simulink model "dspddc"  (Simulink 8.3)
settings: Solver=FixedStepDiscrete  SolverMode=SingleTasking  StartTime=0.0  StopTime=20500/69.333e6  RelTol=1e-3
model workspace (MATLAB code in the model file):
  | gsmcoeffs
libraries: dspmlti4 x4, simulink x2, dspsigops x2, dspsrcs4 x1, dspmisc x1
settings Model: MinMaxOverflowLogging=OverflowOnly  Creator=The MathWorks Inc.  ExtModeAutoUpdateStatusClock=off
settings DataIOCC: LimitDataPoints=off  SaveOutput=off  SaveTime=off  SignalLoggingName=sigsOut
settings OptimizationCC: InlineParams=on  InlineInvariantSignals=on  ExpressionDepthLimit=2147483647  InitFltsAndDblsToZero=on  EfficientMapNaN2IntZero=off
settings DebuggingCC: SaveWithParameterizedLinksMsg=none  CheckExecutionContextPreStartOutputMsg=on  CheckExecutionContextRuntimeOutputMsg=on  SignalResolutionControl=TryResolveAllWithWarning  SolverPrmCheckMsg=none  InheritedTsInSrcMsg=none  MultiTaskDSMMsg=warning  MultiTaskCondExecSysMsg=none  IntegerOverflowMsg=none  ParameterPrecisionLossMsg=none  FcnCallInpInsideContextMsg=UseLocalSettings  StrictBusMsg=None
settings HardwareCC: ProdHWDeviceType=ASIC/FPGA  ProdEqTarget=off
settings RTWCC: IncludeERTFirstTime=on
settings GRTTargetCC: TargetFcnLib=ansi_tfl_tmw.mat

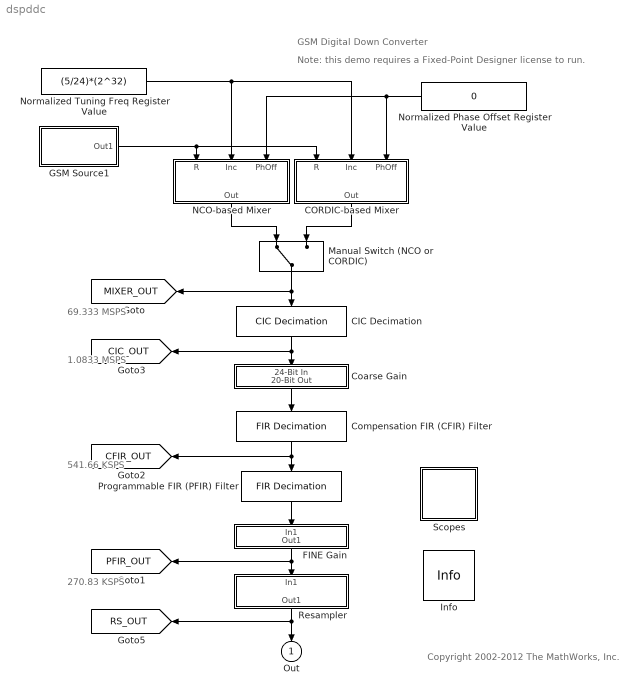
== system dspddc ==
  note: 1.0833
      | MSPS
  note: 541.66
      | KSPS
  note: 270.83
      | KSPS
  note: 69.333
      | MSPS
  note: GSM Digital Down Converter
  note: Note: this demo requires a Fixed-Point Designer license to run.
  note: Copyright 2002-2012 The MathWorks, Inc.
  CIC Decimation : dspmlti4/CIC Decimation  filtFrom=Dialog  filtobj=Hm_decim  ftype=Decimator  R=64  M=1  N=5  filterInternals=Minimum section word lengths  BPS=[50 29 24 24 24 24 24 24 24 24]  FLPS=0  outputWordLength=24  outputFracLength=0  launchFVT=off  framing=Maintain input frame rate  RateOptions=Allow multirate processing
  CORDIC-based Mixer : Subsystem
  Coarse Gain : Subsystem  mask(Coarse Gain){coarse_gain=0}
      mask prompts: coarse_gain "COARSE gain (0-7):"
      mask Help: web(dspdhelp, '-helpbrowser');
      mask Display: disp('Coarse Gain')
  Compensation FIR (CFIR) Filter : dspmlti4/FIR Decimation  h=cfir  D=2  filtStruct=Direct form  framing=Maintain input frame size  inputOffset=0  outputBufInitCond=0  firstCoeffMode=Specify word length  firstCoeffWordLength=16  firstCoeffFracLength=0  firstCoeffDataTypeStr=fixdt(1,16)  firstCoeffLastDataTypeStr=fixdt(1,16)  firstCoeffMin=[]  firstCoeffMax=[]  outputMode=Binary point scaling  outputWordLength=20  outputFracLength=-12  outputDataTypeStr=fixdt(1,20,-12)  outputLastDataTypeStr=fixdt(1,20,-12)  outputMin=[]  outputMax=[]  roundingMode=Floor  overflowMode=off  FilterSource=Specify via dialog  FilterObject=Hm_firdecim
  FINE Gain : Subsystem  mask(Fine Gain){g=1024}
      mask prompts: g "FINE gain (1-16383):"
      mask help: Valid FINE (gain parameter) inputs are positive integers less than 16383. The FINE_GAIN is calculated as FINE/1024.
      mask Help: web(dspdhelp, '-helpbrowser');
      mask Display: disp('Fine Gain')
  GSM Source1 : Subsystem  mask(GSM Source){source_type=Chirp}
      mask prompts: source_type "Source type:"
      mask init:
      | pure_tune_input = (source_type - 1);
      mask Help: web(dspdhelp, '-helpbrowser');
      mask TypeOptions source_type: Chirp | Sinusoid
      mask Display:
      | disp(['GSM' 10 'Source']);
      | 
      | 
      | 
      | 
      | 
      | 
      | port_label('output', 1, 'A/D');
  Info : dspmisc/Info  SystemSampleTime=-1
  Manual Switch (NCO or CORDIC) : ManualSwitch
  NCO-based Mixer : Subsystem
  Normalized Phase Offset Register Value : Constant  Value=0  OutDataTypeStr=int16  SampleTime=-1
  Normalized Tuning Freq Register Value : Constant  Value=(5/24)*(2^32)  OutDataTypeStr=int32
  Programmable FIR (PFIR) Filter : dspmlti4/FIR Decimation  h=pfir  D=2  filtStruct=Direct form  framing=Maintain input frame size  inputOffset=0  outputBufInitCond=0  firstCoeffMode=Specify word length  firstCoeffWordLength=16  firstCoeffFracLength=0  firstCoeffDataTypeStr=fixdt(1,16)  firstCoeffLastDataTypeStr=fixdt(1,16)  firstCoeffMin=[]  firstCoeffMax=[]  outputMode=Binary point scaling  outputWordLength=20  outputFracLength=-12  outputDataTypeStr=fixdt(1,20,-12)  outputLastDataTypeStr=fixdt(1,20,-12)  outputMin=[]  outputMax=[]  roundingMode=Floor  overflowMode=off  FilterSource=Specify via dialog  FilterObject=Hm_firdecim
  Resampler : Subsystem  mask(Resampler){h=fir1(31,0.25), Ndelay=4, Ndec=3}
      mask prompts: h "Resampling FIR coefficients:"; Ndelay "NDELAY (upsample factor):"; Ndec "NDEC (downsample factor):"
      mask Help: web(dspdhelp, '-helpbrowser');
      mask Display: disp('Rate Conversion')
  Scopes : Subsystem
      mask Display: disp('Scopes')
  Out : Outport
  tag scope: CFIR_OUT=global, CIC_OUT=global, MIXER_OUT=global, PFIR_OUT=global, RS_OUT=global
  wires:
  Compensation FIR (CFIR) Filter/1 -> [CFIR_OUT], Programmable FIR (PFIR) Filter/1
  Programmable FIR (PFIR) Filter/1 -> FINE Gain/1(In1)
  Resampler/1(Out1) -> Out/1, [RS_OUT]
  CIC Decimation/1 -> Coarse Gain/1(24-Bit In), [CIC_OUT]
  Coarse Gain/1(20-Bit Out) -> Compensation FIR (CFIR) Filter/1
  FINE Gain/1(Out1) -> Resampler/1(In1), [PFIR_OUT]
  GSM Source1/1(Out1) -> NCO-based Mixer/1(R), CORDIC-based Mixer/1(R)
  Normalized Tuning Freq Register Value/1 -> NCO-based Mixer/2(Inc), CORDIC-based Mixer/2(Inc)
  NCO-based Mixer/1(Out) -> Manual Switch (NCO or CORDIC)/1
  Normalized Phase Offset Register Value/1 -> NCO-based Mixer/3(PhOff), CORDIC-based Mixer/3(PhOff)
  CORDIC-based Mixer/1(Out) -> Manual Switch (NCO or CORDIC)/2
  Manual Switch (NCO or CORDIC)/1 -> CIC Decimation/1, [MIXER_OUT]

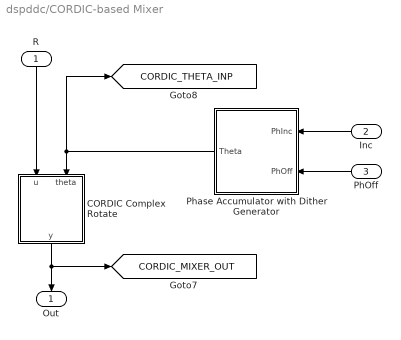
== system dspddc/CORDIC-based Mixer ==
  R : Inport
  Inc : Inport  Port=2
  PhOff : Inport  Port=3
  CORDIC Complex Rotate : MATLAB Function  TreatAsAtomicUnit=on
  Phase Accumulator with Dither Generator : Subsystem
  Out : Outport
  tag scope: CORDIC_MIXER_OUT=global, CORDIC_THETA_INP=global
  wires:
  Inc/1 -> Phase Accumulator with Dither Generator/1(PhInc)
  R/1 -> CORDIC Complex Rotate/1(u)
  CORDIC Complex Rotate/1(y) -> Out/1, [CORDIC_MIXER_OUT]
  Phase Accumulator with Dither Generator/1(Theta) -> CORDIC Complex Rotate/2(theta), [CORDIC_THETA_INP]
  PhOff/1 -> Phase Accumulator with Dither Generator/2(PhOff)

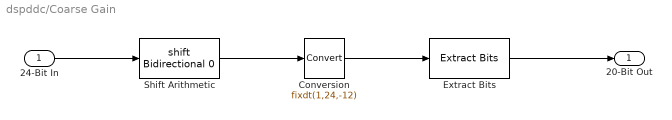
== system dspddc/Coarse Gain ==
  24-Bit In : Inport
  Conversion : DataTypeConversion  OutDataTypeStr=fixdt(1,24,-12)  SaturateOnIntegerOverflow=on
  Extract Bits : simulink/Logic and Bit Operations/Extract Bits  bitsToExtract=Range of bits  numBits=8  bitIdxRange=[0 19]  outScalingMode=Preserve fixed-point scaling
  Shift Arithmetic : ArithShift
  20-Bit Out : Outport
  wires:
  Shift Arithmetic/1 -> Conversion/1
  24-Bit In/1 -> Shift Arithmetic/1
  Extract Bits/1 -> 20-Bit Out/1
  Conversion/1 -> Extract Bits/1

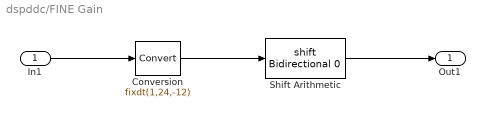
== system dspddc/FINE Gain ==
  In1 : Inport
  Conversion : DataTypeConversion  OutDataTypeStr=fixdt(1,24,-12)  SaturateOnIntegerOverflow=on
  Shift Arithmetic : ArithShift
  Out1 : Outport
  wires:
  Conversion/1 -> Shift Arithmetic/1
  In1/1 -> Conversion/1
  Shift Arithmetic/1 -> Out1/1

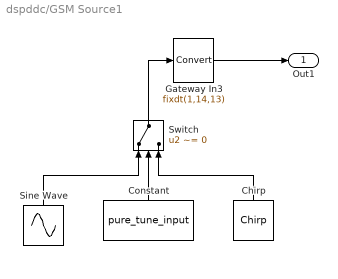
== system dspddc/GSM Source1 ==
  Chirp : dspsrcs4/Chirp  sweep=Linear  mode=Unidirectional  f0=.2078*69.333e6  f1=.2088*69.333e6  t1=16384/69.333e6  Tsweep=16384/69.333e6  phase=0  Ts=1/69.333e6  spf=1  datatype=Double
  Constant : Constant  Value=pure_tune_input  OutDataTypeStr=boolean
  Gateway In3 : DataTypeConversion  OutDataTypeStr=fixdt(1,14,13)  RndMeth=Nearest  SaturateOnIntegerOverflow=on
  Sine Wave : Sin  Frequency=2*pi*69.1e6*5/24  SampleTime=1/69.333e6
  Switch : Switch  Criteria=u2 ~= 0  Threshold=0.5  InputSameDT=on
  Out1 : Outport
  wires:
  Switch/1 -> Gateway In3/1
  Sine Wave/1 -> Switch/1
  Chirp/1 -> Switch/3
  Constant/1 -> Switch/2
  Gateway In3/1 -> Out1/1

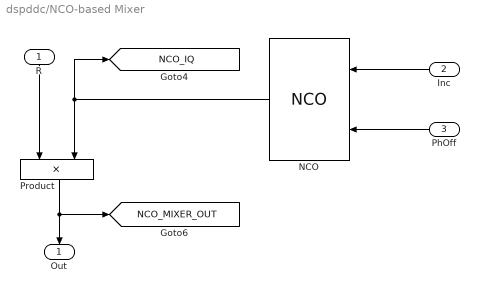
== system dspddc/NCO-based Mixer ==
  R : Inport
  Inc : Inport  Port=2
  PhOff : Inport  Port=3
  NCO : dspsigops/NCO  AccIncSrc=Input port  AccInc=100  PhaseOffsetSrc=Input port  PhaseOffset=0  AccumWL=32  HasDither=on  DitherWL=15  PNgeneratorLength=12  HasPhaseQuantizer=on  TableDepth=18  HasOutputPhaseError=off  Formula=Complex exponential  DataType=Binary point scaling  OutputWL=20  OutputFL=18  CompMethod=Table lookup (no interpolation)  SampleTime=1  SamplesPerFrame=1
  Product : Product  OutDataTypeStr=fixdt(1,20,18)  RndMeth=Nearest
  Out : Outport
  tag scope: NCO_IQ=global, NCO_MIXER_OUT=global
  wires:
  NCO/1 -> Product/2, [NCO_IQ]
  PhOff/1 -> NCO/2
  R/1 -> Product/1
  Inc/1 -> NCO/1
  Product/1 -> Out/1, [NCO_MIXER_OUT]

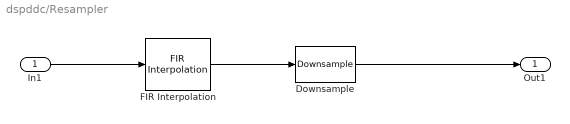
== system dspddc/Resampler ==
  In1 : Inport
  Downsample : dspsigops/Downsample  N=Ndec  phase=0  RateOptions=Allow multirate processing  smode=Allow multirate  fmode=Maintain input frame size  ic=0
  FIR Interpolation : dspmlti4/FIR Interpolation  h=h  L=Ndelay  framing=Maintain input frame size  outputBufInitCond=0  firstCoeffMode=Specify word length  firstCoeffWordLength=12  firstCoeffFracLength=0  firstCoeffDataTypeStr=fixdt(1,12)  firstCoeffLastDataTypeStr=fixdt(1,12)  firstCoeffMin=[]  firstCoeffMax=[]  outputMode=Binary point scaling  outputWordLength=24  outputFracLength=-12  outputDataTypeStr=fixdt(1,24,-12)  outputLastDataTypeStr=fixdt(1,24,-12)  outputMin=[]  outputMax=[]  roundingMode=Floor  overflowMode=off  FilterSource=Specify via dialog  FilterObject=Hm_firinterp
  Out1 : Outport
  wires:
  In1/1 -> FIR Interpolation/1
  Downsample/1 -> Out1/1
  FIR Interpolation/1 -> Downsample/1

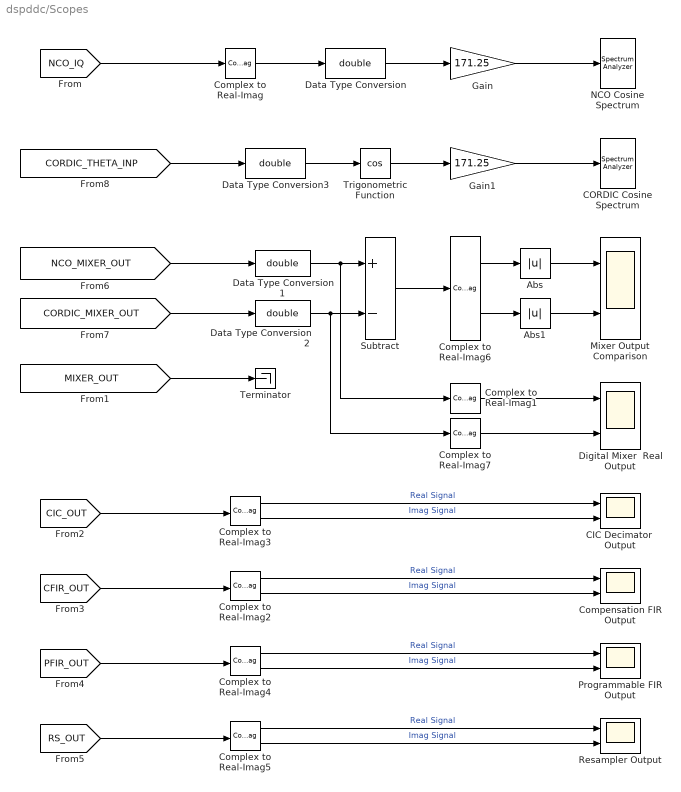
== system dspddc/Scopes ==
  Abs : Abs
  Abs1 : Abs
  CIC Decimator  Output : Scope  NumInputPorts=2
      settings: TimeRange=0.0003  YMin=-1e+009~-1e+009  YMax=1e+009~1e+009  DataFormat=Structure  MaxDataPoints=1000000
  CORDIC Cosine Spectrum : SpectrumAnalyzer  ScopeSpecification=DataTag6
  Compensation FIR Output : Scope  NumInputPorts=2
      settings: TimeRange=0.0003  YMin=-1e+009~-1e+009  YMax=1e+009~1e+009  SaveName=ScopeData2  DataFormat=Structure  MaxDataPoints=1000000
  Complex to Real-Imag : ComplexToRealImag  Output=Real
  Complex to Real-Imag1 : ComplexToRealImag  Output=Real
  Complex to Real-Imag{2..6} (5 alike) : ComplexToRealImag
  Complex to Real-Imag7 : ComplexToRealImag  Output=Real
  Data Type Conversion : DataTypeConversion  OutDataTypeStr=double  SaturateOnIntegerOverflow=on  RndMeth=Zero
  Data Type Conversion1 : DataTypeConversion  OutDataTypeStr=double
  Data Type Conversion2 : DataTypeConversion  OutDataTypeStr=double
  Data Type Conversion3 : DataTypeConversion  OutDataTypeStr=double  SaturateOnIntegerOverflow=on  RndMeth=Zero
  Digital Mixer  Real Output : Scope  NumInputPorts=2
      settings: TimeRange=0.0003  YMin=-1~-1  YMax=1~1  SaveName=ScopeData5  DataFormat=Structure  MaxDataPoints=1000000
  Gain : Gain  Gain=171.25  SaturateOnIntegerOverflow=on  OutDataTypeStr=Inherit: Same as input  ParamDataTypeStr=Inherit: Same as input
  Gain1 : Gain  Gain=171.25  SaturateOnIntegerOverflow=on  OutDataTypeStr=Inherit: Same as input  ParamDataTypeStr=Inherit: Same as input
  Mixer Output Comparison : Scope  NumInputPorts=2
      settings: TimeRange=0.0003  YMin=0~0  YMax=0.001~0.001  DataFormat=Structure  MaxDataPoints=1000000
  NCO Cosine Spectrum : SpectrumAnalyzer  ScopeSpecification=DataTag7
  Programmable FIR Output : Scope  NumInputPorts=2
      settings: TimeRange=0.0003  YMin=-1000000000~-1000000000  YMax=1000000000~1000000000  SaveName=ScopeData3  DataFormat=Structure  MaxDataPoints=1000000
  Resampler Output : Scope  NumInputPorts=2
      settings: TimeRange=0.0003  YMin=-200000000~-200000000  YMax=200000000~200000000  SaveName=ScopeData4  DataFormat=Structure  MaxDataPoints=1000000
  Subtract : Sum  Inputs=+-  OutDataTypeStr=Inherit: Same as accumulator
  Terminator : Terminator
  Trigonometric Function : Trigonometry  Operator=cos
  wires:
  Complex to Real-Imag/1 -> Data Type Conversion/1
  Gain/1 -> NCO Cosine Spectrum/1
  [NCO_IQ] -> Complex to Real-Imag/1
  Data Type Conversion/1 -> Gain/1
  [MIXER_OUT] -> Terminator/1
  Complex to Real-Imag3/1 -> CIC Decimator  Output/1  "Real Signal"
  Complex to Real-Imag3/2 -> CIC Decimator  Output/2  "Imag Signal"
  [CIC_OUT] -> Complex to Real-Imag3/1
  Complex to Real-Imag2/1 -> Compensation FIR Output/1  "Real Signal"
  Complex to Real-Imag2/2 -> Compensation FIR Output/2  "Imag Signal"
  [CFIR_OUT] -> Complex to Real-Imag2/1
  Complex to Real-Imag4/1 -> Programmable FIR Output/1  "Real Signal"
  Complex to Real-Imag4/2 -> Programmable FIR Output/2  "Imag Signal"
  [PFIR_OUT] -> Complex to Real-Imag4/1
  Complex to Real-Imag5/1 -> Resampler Output/1  "Real Signal"
  Complex to Real-Imag5/2 -> Resampler Output/2  "Imag Signal"
  [RS_OUT] -> Complex to Real-Imag5/1
  Subtract/1 -> Complex to Real-Imag6/1
  Complex to Real-Imag6/1 -> Abs/1
  Complex to Real-Imag6/2 -> Abs1/1
  [NCO_MIXER_OUT] -> Data Type Conversion1/1
  [CORDIC_MIXER_OUT] -> Data Type Conversion2/1
  Abs/1 -> Mixer Output Comparison/1
  Abs1/1 -> Mixer Output Comparison/2
  Data Type Conversion1/1 -> Subtract/1, Complex to Real-Imag1/1
  Data Type Conversion2/1 -> Subtract/2, Complex to Real-Imag7/1
  [CORDIC_THETA_INP] -> Data Type Conversion3/1
  Data Type Conversion3/1 -> Trigonometric Function/1
  Trigonometric Function/1 -> Gain1/1
  Gain1/1 -> CORDIC Cosine Spectrum/1
  Complex to Real-Imag1/1 -> Digital Mixer  Real Output/1
  Complex to Real-Imag7/1 -> Digital Mixer  Real Output/2

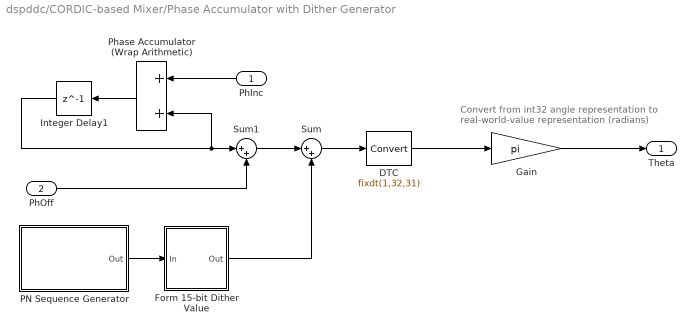
== system dspddc/CORDIC-based Mixer/Phase Accumulator with Dither Generator ==
  note: Convert from int32 angle representation
      | to real-world-value representation (radians)
  PhInc : Inport
  PhOff : Inport  Port=2
  DTC : DataTypeConversion  OutDataTypeStr=fixdt(1,32,31)  ConvertRealWorld=Stored Integer (SI)
  Form 15-bit Dither Value : Subsystem
  Gain : Gain  Gain=pi  ParamDataTypeStr=fixdt(1,20)  OutDataTypeStr=fixdt(1,20,17)
  Integer Delay1 : Delay  DelayLength=1  InputProcessing=Inherited
  PN Sequence Generator : Subsystem
  Phase Accumulator (Wrap Arithmetic) : Sum  InputSameDT=on  OutDataTypeStr=Inherit: Same as first input
  Sum : Sum  Inputs=|++  OutDataTypeStr=Inherit: Same as accumulator
  Sum1 : Sum  Inputs=|++  OutDataTypeStr=Inherit: Same as accumulator
  Theta : Outport
  wires:
  Phase Accumulator (Wrap Arithmetic)/1 -> Integer Delay1/1
  PhInc/1 -> Phase Accumulator (Wrap Arithmetic)/1
  DTC/1 -> Gain/1
  Gain/1 -> Theta/1
  Integer Delay1/1 -> Phase Accumulator (Wrap Arithmetic)/2, Sum1/1
  Sum/1 -> DTC/1
  PN Sequence Generator/1(Out) -> Form 15-bit Dither Value/1(In)
  Form 15-bit Dither Value/1(Out) -> Sum/2
  Sum1/1 -> Sum/1
  PhOff/1 -> Sum1/2

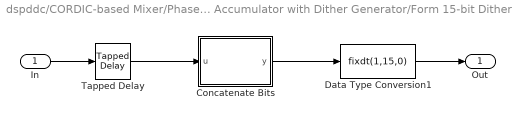
== system dspddc/CORDIC-based Mixer/Phase Accumulator with Dither Generator/Form 15-bit Dither Value ==
  In : Inport
  Concatenate Bits : MATLAB Function  TreatAsAtomicUnit=on
  Data Type Conversion1 : DataTypeConversion  OutDataTypeStr=fixdt(1,15,0)  ConvertRealWorld=Stored Integer (SI)
  Tapped Delay : simulink/Discrete/Tapped Delay  vinit=1  samptime=-1  NumDelays=14  DelayOrder=Oldest  includeCurrent=on
  Out : Outport
  wires:
  Tapped Delay/1 -> Concatenate Bits/1(u)
  Concatenate Bits/1(y) -> Data Type Conversion1/1
  Data Type Conversion1/1 -> Out/1
  In/1 -> Tapped Delay/1

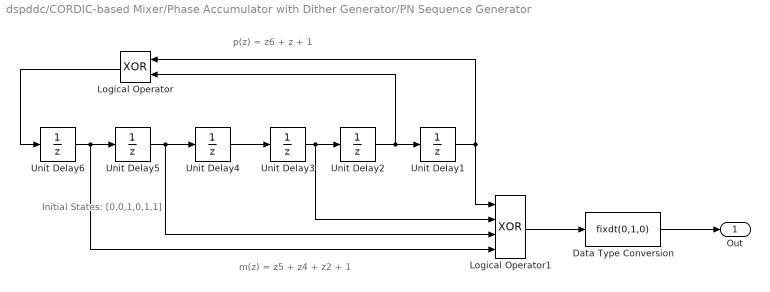
== system dspddc/CORDIC-based Mixer/Phase Accumulator with Dither Generator/PN Sequence Generator ==
  note: p(z) = z6 + z + 1
  note: m(z) = z5 + z4 + z2 + 1
  note: Initial States:
      | [0,0,1,0,1,1]
  Data Type Conversion : DataTypeConversion  OutDataTypeStr=fixdt(0,1,0)
  Logical Operator : Logic  Operator=XOR  AllPortsSameDT=off  OutDataTypeStr=boolean
  Logical Operator1 : Logic  Operator=XOR  Inputs=4  AllPortsSameDT=off  OutDataTypeStr=boolean
  Unit Delay1 : UnitDelay  InitialCondition=1  SampleTime=-1
  Unit Delay2 : UnitDelay  InitialCondition=1  SampleTime=-1
  Unit Delay3 : UnitDelay  SampleTime=-1
  Unit Delay4 : UnitDelay  InitialCondition=1  SampleTime=-1
  Unit Delay5 : UnitDelay  SampleTime=-1
  Unit Delay6 : UnitDelay  SampleTime=-1
  Out : Outport
  wires:
  Logical Operator/1 -> Unit Delay6/1
  Unit Delay6/1 -> Unit Delay5/1, Logical Operator1/4
  Unit Delay5/1 -> Unit Delay4/1, Logical Operator1/3
  Unit Delay4/1 -> Unit Delay3/1
  Unit Delay3/1 -> Unit Delay2/1, Logical Operator1/2
  Unit Delay2/1 -> Unit Delay1/1, Logical Operator/2
  Unit Delay1/1 -> Logical Operator1/1, Logical Operator/1
  Logical Operator1/1 -> Data Type Conversion/1
  Data Type Conversion/1 -> Out/1

== matlab function CORDIC-based Mixer/Phase Accumulator with Dither Generator/Form 15-bit Dither Value/Concatenate Bits ==
  data: u input double; y output double
function y = fcn(u)
% Concatenate bits in a quasi-random permuted order
y = bitconcat(u(1),u(7),u(11),u(5),u(15),u(3),u(13),u(9),...
    u(2),u(4),u(14),u(8),u(12),u(10),u(6));

== matlab function CORDIC-based Mixer/CORDIC Complex Rotate ==
  data: u input double; y output double; theta input double
function y = fcn(u, theta)
niters = 15; % Number of CORDIC iterations
y      = cordicrotate(theta, u, niters);
